simulink model "Prodline_EF_RL"  (R2023b)
settings: Solver=VariableStepDiscrete  StartTime=0  StopTime=Inf  RelTol=1e-3
model workspace (MAT data in the model file):
  EpisodeData.ExplorationProbability = 0.01
  EpisodeData.LearnRate = 0.7
  EpisodeData.DiscountFactor = 0.9
  EpisodeData.Table = [32.3279808057 48.3662273221 56.8010564606 75.8199870142 94.2467100891 126.392175074 147.868902265 201.713499215 225.197534088 273.928372258 470.902807484 558.602771343 ... (3844 elements, 1922x2)]
  EpisodeData.TotalReward = 0
  EpisodeData.LastEpisode = 0
  EpisodeData.Seed = 20000
  SimOptions.tMax = 480
  SimOptions.ProcessingTime_Job1 = 1
  SimOptions.ProcessingTime_Job2 = 3
  SimOptions.RetoolingTime = 3
  SimOptions.SaleTime_Job1 = 10
  SimOptions.SaleTime_Job2 = 5
  SimOptions.MaxQueueLength = 30
  SimOptions.MaxDeltaQueue = 10
undefined symbols (not defined in the file or in its folder): i, m, n
libraries: simulink x1, rllib x1
settings Model: SimulationMode=accelerator  Creator=jan  LastModifiedBy=jan
settings SolverCC: AllowMultiTaskInputOutput=on
settings OptimizationCC: ReuseModelBlockBuffer=off
settings ModelReferenceCC: EnableRefExpFcnMdlSchedulingChecks=on

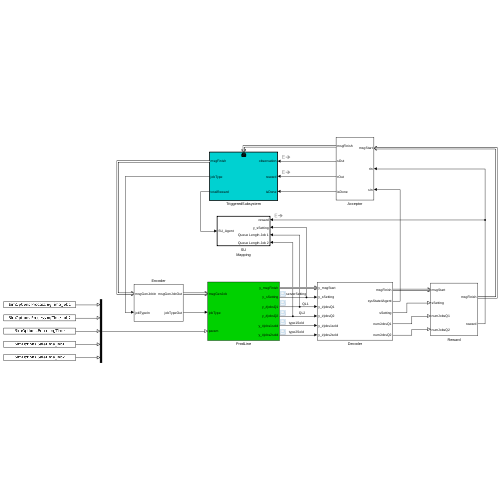
[thumbnail: Simulink's stored preview of the top-level diagram]
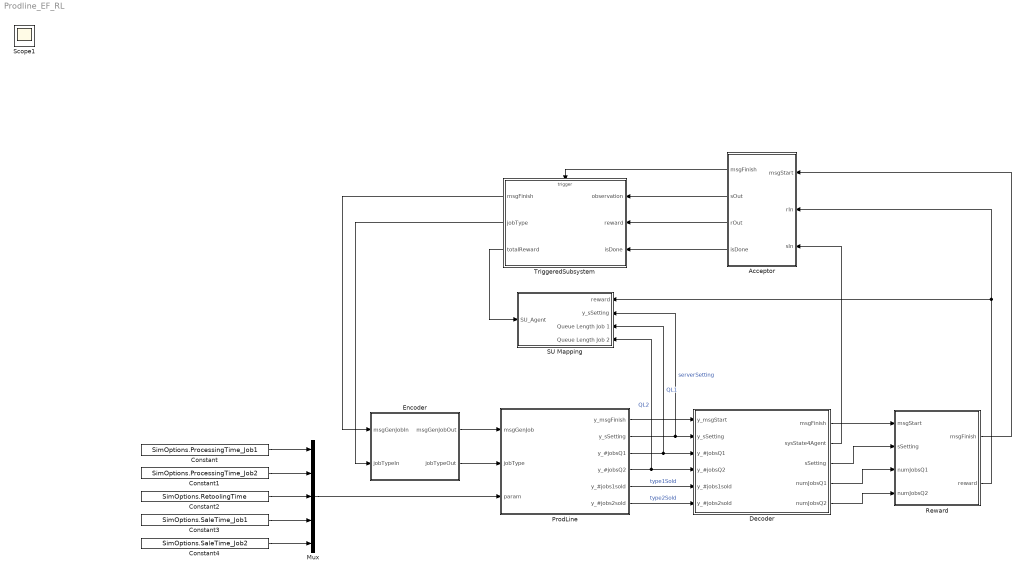
== system Prodline_EF_RL ==
  Acceptor : Subsystem
  Constant : Constant  Value=SimOptions.ProcessingTime_Job1
  Constant1 : Constant  Value=SimOptions.ProcessingTime_Job2
  Constant2 : Constant  Value=SimOptions.RetoolingTime
  Constant3 : Constant  Value=SimOptions.SaleTime_Job1
  Constant4 : Constant  Value=SimOptions.SaleTime_Job2
  Decoder : Subsystem
  Encoder : Subsystem
  Mux : Mux  Inputs=5
  ProdLine : Subsystem
  Reward : Subsystem
  SU Mapping : Subsystem  TreatAsAtomicUnit=on
      settings: PortSchema="{\"entries\":[{\"content\":{\"sides\":[{\"content\":{\"connectorIds\":[\"In1\",\"In2\",\"In3\",\"In4\"]},\"type\":\"ConnectorPlacement.EquallySpacedRectSide\",\"uuid\":\"25726879-9920-47f0-bc13-fe4ee4fad127\"},{\"content\":{\"connectorIds\":[\"In5\"],\"side\":\"RIGHT\"},\"type\":\"ConnectorPlacement.EquallySpacedRectSide\",\"uuid\":\"76e5ad88-c4d3-414b-b9a6-05d87e69b074\"},{\"content\":{\"connectorIds\":[],\"side\":\"TOP\"},\"type\":\"ConnectorPlacement.EquallySpacedRectSide\",\"uuid\":\"0e81be63-41e4-4d16-953c-cb60ef6ef114\"}]},\"type\":\"ConnectorPlacement.EquallySpacedConnector\",\"uuid\":\"9bcce8c0-ed31-4d29-947b-6e1387c3e550\"}],\"packageUris\":[\"http://schema.mathworks.com/mf0/Connector/R2020b\"],\"version\":\"1.0\"}"
  TriggeredSubsystem : Subsystem  InputPortMessageModes=i,i,i,m  TreatAsAtomicUnit=on
  Scope1 : Scope
  wires:
  Mux/1 -> ProdLine/3(param)
  Constant/1 -> Mux/1
  Constant1/1 -> Mux/2
  Constant2/1 -> Mux/3
  Constant3/1 -> Mux/4
  Constant4/1 -> Mux/5
  Encoder/1(msgGenJobOut) -> ProdLine/1(msgGenJob)
  Encoder/2(jobTypeOut) -> ProdLine/2(jobType)
  ProdLine/2(y_sSetting) -> Decoder/2(y_sSetting), SU Mapping/2(y_sSetting)  "serverSetting"
  ProdLine/3(y_#jobsQ1) -> SU Mapping/3(Queue Length Job 1), Decoder/3(y_#jobsQ1)  "QL1"
  ProdLine/4(y_#jobsQ2) -> Decoder/4(y_#jobsQ2), SU Mapping/4(Queue Length Job 2)  "QL2"
  ProdLine/5(y_#jobs1sold) -> Decoder/5(y_#jobs1sold)  "type1Sold"
  ProdLine/6(y_#jobs2sold) -> Decoder/6(y_#jobs2sold)  "type2Sold"
  Decoder/1(msgFinish) -> Reward/1(msgStart)
  ProdLine/1(y_msgFinish) -> Decoder/1(y_msgStart)
  Decoder/3(sSetting) -> Reward/2(sSetting)
  Decoder/4(numJobsQ1) -> Reward/3(numJobsQ1)
  Decoder/5(numJobsQ2) -> Reward/4(numJobsQ2)
  Decoder/2(sysState4Agent) -> Acceptor/3(sIn)
  Reward/1(msgFinish) -> Acceptor/1(msgStart)
  Reward/2(reward) -> SU Mapping/1(reward), Acceptor/2(rIn)
  Acceptor/3(rOut) -> TriggeredSubsystem/2(reward)
  Acceptor/4(isDone) -> TriggeredSubsystem/3(isDone)
  Acceptor/1(msgFinish) -> TriggeredSubsystem/Trigger
  TriggeredSubsystem/1(msgFinish) -> Encoder/1(msgGenJobIn)
  TriggeredSubsystem/2(jobType) -> Encoder/2(jobTypeIn)
  TriggeredSubsystem/3(totalReward) -> SU Mapping/5(SU_Agent)
  Acceptor/2(sOut) -> TriggeredSubsystem/1(observation)

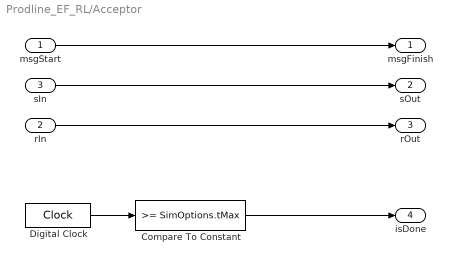
== system Prodline_EF_RL/Acceptor ==
  msgStart : Inport
  rIn : Inport  Port=2
  sIn : Inport  Port=3
  Compare To Constant : simulink/Logic and Bit Operations/Compare To Constant  relop=>=  const=SimOptions.tMax  OutDataTypeStr=boolean  ZeroCross=off
  Digital Clock : DigitalClock
  msgFinish : Outport
  sOut : Outport  Port=2
  rOut : Outport  Port=3
  isDone : Outport  Port=4
  wires:
  Digital Clock/1 -> Compare To Constant/1
  sIn/1 -> sOut/1
  msgStart/1 -> msgFinish/1
  rIn/1 -> rOut/1
  Compare To Constant/1 -> isDone/1

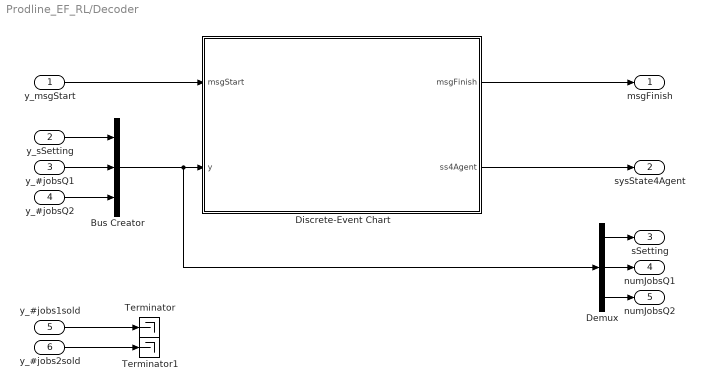
== system Prodline_EF_RL/Decoder ==
  y_msgStart : Inport
  y_sSetting : Inport  Port=2
  y_#jobsQ1 : Inport  Port=3
  y_#jobsQ2 : Inport  Port=4
  y_#jobs1sold : Inport  Port=5
  y_#jobs2sold : Inport  Port=6
  Bus Creator : BusCreator  Inputs=3
  Demux : Demux  Outputs=3
  Discrete-Event Chart : Stateflow chart  TreatAsAtomicUnit=on
  Terminator : Terminator
  Terminator1 : Terminator
  msgFinish : Outport
  sysState4Agent : Outport  Port=2  OutDataTypeStr=uint32
  sSetting : Outport  Port=3
  numJobsQ1 : Outport  Port=4
  numJobsQ2 : Outport  Port=5
  wires:
  Discrete-Event Chart/2(ss4Agent) -> sysState4Agent/1
  Bus Creator/1 -> Demux/1, Discrete-Event Chart/2(y)
  y_sSetting/1 -> Bus Creator/1
  y_#jobsQ1/1 -> Bus Creator/2
  y_#jobsQ2/1 -> Bus Creator/3
  Discrete-Event Chart/1(msgFinish) -> msgFinish/1
  y_#jobs1sold/1 -> Terminator/1
  y_#jobs2sold/1 -> Terminator1/1
  Demux/2 -> numJobsQ1/1
  Demux/1 -> sSetting/1
  Demux/3 -> numJobsQ2/1
  y_msgStart/1 -> Discrete-Event Chart/1(msgStart)

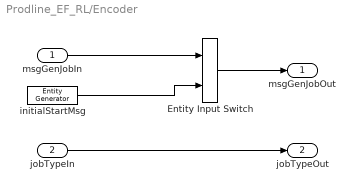
== system Prodline_EF_RL/Encoder ==
  msgGenJobIn : Inport
  jobTypeIn : Inport  Port=2
  Entity Input Switch : EntityInputSwitch  InputPortMessageModes=m,m  OutputPortMessageModes=m
  initialStartMsg : EntityGenerator  OutputPortMessageModes=m  Period=Inf  AttributeName=entity  EntityTypeName=Entity  DataInitialValue=1
  msgGenJobOut : Outport
  jobTypeOut : Outport  Port=2
  wires:
  msgGenJobIn/1 -> Entity Input Switch/1
  initialStartMsg/1 -> Entity Input Switch/2
  Entity Input Switch/1 -> msgGenJobOut/1
  jobTypeIn/1 -> jobTypeOut/1

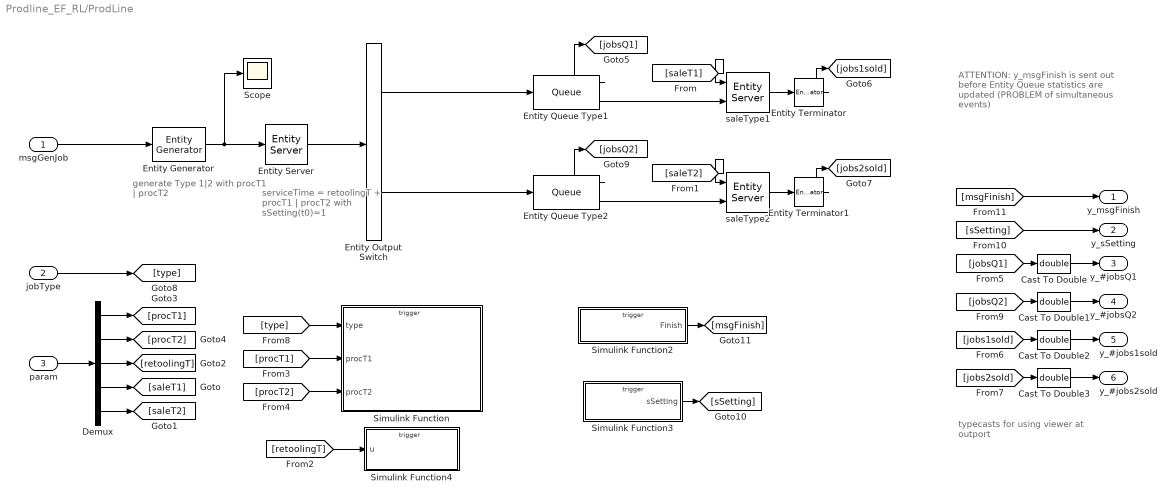
== system Prodline_EF_RL/ProdLine ==
  note: generate Type 1|2
      | with procT1 | procT2
  note: ATTENTION:
      | y_msgFinish is sent out
      | before Entity Queue
      | statistics are updated
      | (PROBLEM of
      | simultaneous events)
  note: serviceTime =
      | retoolingT +
      | procT1 | procT2
      |      with
      | sSetting(t0)=1
  note: typecasts for using
      | viewer at outport
  msgGenJob : Inport
  jobType : Inport  Port=2
  param : Inport  Port=3
  Cast To Double{,1..3} (4 alike) : DataTypeConversion  OutDataTypeStr=double  SaturateOnIntegerOverflow=off  RndMeth=Floor
  Demux : Demux  Outputs=5
  Entity Output Switch : EntityOutputSwitch  InputPortMessageModes=m  OutputPortMessageModes=m,m  SwitchingCriterion=From attribute  SwitchAttributeName=Type
  Entity Generator : EntityGenerator  InputPortMessageModes=m  OutputPortMessageModes=m  GenerationMethod=Event-based  GenerateAction=|  AttributeName=ID|Type|ProcessingTime|ServiceTime  AttributeInitialValue=1|0|0|0  EntityType=Structured  EntityTypeName=Job
      | % Use a persistent counter to set ID
      | persistent next_id
      | if isempty(next_id)
      |     next_id = 1;
      |     %{
      |     % IS NOT Necessary!
      |     % Set seed for random number generator
      |     rng(12345)
      |     %}
      | end
      | 
      | % Assign ID attribute
      | entity.ID = next_id;
      | next_id = next_id +1;
      | 
      | %Assign job Type and ProcessingTime
      | %entity.Type = setJobType()
      | [entity.Type,entity.ProcessingTime]=setAttributes();
      settings: InputPortMap=u0
  Entity Queue Type1 : Queue  InputPortMessageModes=m  OutputPortMessageModes=n,m  Capacity=Inf  EntryAction=|  NumberEntitiesInBlock=on
      | % Generate finish msg
      | sendFinish(entity.Type)
      settings: OutputPortMap=o1,o5
  Entity Queue Type2 : Queue  InputPortMessageModes=m  OutputPortMessageModes=n,m  Capacity=Inf  EntryAction=|  NumberEntitiesInBlock=on
      | % Generate finish msg
      | sendFinish(entity.Type);
      settings: OutputPortMap=o1,o5
  Entity Server : EntityServer  InputPortMessageModes=m  OutputPortMessageModes=m  Capacity=1  ServiceTimeSource=Attribute  EntryAction=|  ExitAction=|
      EntryAction=|
      | % Use a persistent var to store the current server setting
      | % server setting is 1 | 2
      | persistent serverSetting
      | if isempty(serverSetting)
      |     serverSetting = 1;     % init serverSetting
      | end
      | 
      | % Test if new serverSetting is necessary (retooling)
      | if serverSetting ~= entity.Type
      |    entity.ServiceTime = entity.ProcessingTime + retoolingTime();
      |    serverSetting = entity.Type;
      | else
      |     entity.ServiceTime = entity.ProcessingTime;
      | end
      | 
      | % Output current serverSetting
      | outServerSetting(serverSetting)
      ExitAction=|
      | % Generate finish msg
      | %sendFinish();
  Entity Terminator : EntityTerminator  InputPortMessageModes=m  NumberEntitiesArrived=on
      settings: OutputPortMap=o0
  Entity Terminator1 : EntityTerminator  InputPortMessageModes=m  NumberEntitiesArrived=on
      settings: OutputPortMap=o0
  Scope : Scope
  Simulink Function : Subsystem  TreatAsAtomicUnit=on
  Simulink Function2 : Subsystem  TreatAsAtomicUnit=on
  Simulink Function3 : Subsystem  TreatAsAtomicUnit=on
  Simulink Function4 : Subsystem  TreatAsAtomicUnit=on
  saleType1 : EntityServer  InputPortMessageModes=n,m  OutputPortMessageModes=m  Capacity=1  ServiceTimeSource=Signal port  ServiceTimeValue=10
      settings: InputPortMap=u0,u2
  saleType2 : EntityServer  InputPortMessageModes=n,m  OutputPortMessageModes=m  Capacity=1  ServiceTimeSource=Signal port  ServiceTimeValue=5
      settings: InputPortMap=u0,u2
  y_msgFinish : Outport
  y_sSetting : Outport  Port=2
  y_#jobsQ1 : Outport  Port=3
  y_#jobsQ2 : Outport  Port=4
  y_#jobs1sold : Outport  Port=5
  y_#jobs2sold : Outport  Port=6
  wires:
  Simulink Function2/1(" Finish") -> [msgFinish]
  [procT2] -> Simulink Function/3(procT2)
  Demux/5 -> [saleT2]
  Entity Terminator1/1 -> [jobs2sold]
  Entity Output Switch/1 -> Entity Queue Type1/1
  [jobs2sold] -> Cast To Double3/1
  Demux/2 -> [procT2]
  Simulink Function3/1(sSetting) -> [sSetting]
  Cast To Double2/1 -> y_#jobs1sold/1
  [saleT1] -> saleType1/1
  [jobsQ2] -> Cast To Double1/1
  [retoolingT] -> Simulink Function4/1(u)
  Cast To Double3/1 -> y_#jobs2sold/1
  [type] -> Simulink Function/1(type)
  [msgFinish] -> y_msgFinish/1
  Entity Server/1 -> Entity Output Switch/1
  Entity Generator/1 -> Scope/1, Entity Server/1
  Demux/1 -> [procT1]
  Entity Output Switch/2 -> Entity Queue Type2/1
  jobType/1 -> [type]
  param/1 -> Demux/1
  Demux/4 -> [saleT1]
  Entity Terminator/1 -> [jobs1sold]
  [procT1] -> Simulink Function/2(procT1)
  Cast To Double1/1 -> y_#jobsQ2/1
  msgGenJob/1 -> Entity Generator/1
  Entity Queue Type2/2 -> saleType2/2
  [jobsQ1] -> Cast To Double/1
  Entity Queue Type1/2 -> saleType1/2
  Demux/3 -> [retoolingT]
  Entity Queue Type1/1 -> [jobsQ1]
  Cast To Double/1 -> y_#jobsQ1/1
  [saleT2] -> saleType2/1
  [sSetting] -> y_sSetting/1
  saleType1/1 -> Entity Terminator/1
  Entity Queue Type2/1 -> [jobsQ2]
  saleType2/1 -> Entity Terminator1/1
  [jobs1sold] -> Cast To Double2/1

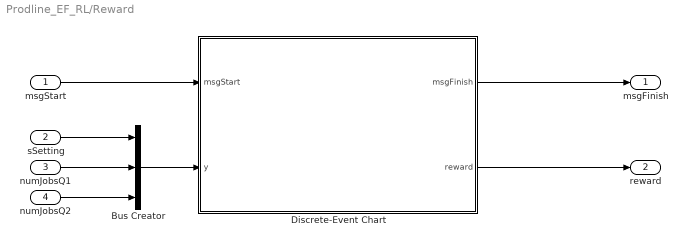
== system Prodline_EF_RL/Reward ==
  msgStart : Inport
  sSetting : Inport  Port=2
  numJobsQ1 : Inport  Port=3
  numJobsQ2 : Inport  Port=4
  Bus Creator : BusCreator  Inputs=3
  Discrete-Event Chart : Stateflow chart  TreatAsAtomicUnit=on
  msgFinish : Outport
  reward : Outport  Port=2
  wires:
  Discrete-Event Chart/1(msgFinish) -> msgFinish/1
  msgStart/1 -> Discrete-Event Chart/1(msgStart)
  Discrete-Event Chart/2(reward) -> reward/1
  Bus Creator/1 -> Discrete-Event Chart/2(y)
  numJobsQ1/1 -> Bus Creator/2
  sSetting/1 -> Bus Creator/1
  numJobsQ2/1 -> Bus Creator/3

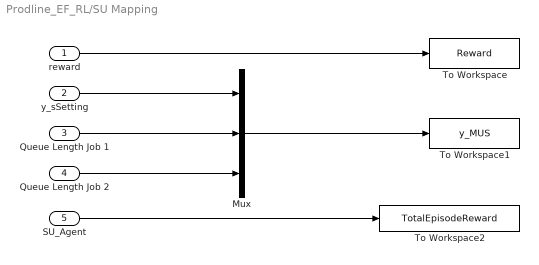
== system Prodline_EF_RL/SU Mapping ==
  reward : Inport
  y_sSetting : Inport  Port=2
  Queue Length Job 1 : Inport  Port=3
  Queue Length Job 2 : Inport  Port=4
  SU_Agent : Inport  Port=5
  Mux : Mux  Inputs=3
  To Workspace : ToWorkspace  VariableName=Reward  SaveFormat=Timeseries  SampleTime=-1
  To Workspace1 : ToWorkspace  VariableName=y_MUS  SaveFormat=Timeseries  SampleTime=-1
  To Workspace2 : ToWorkspace  VariableName=TotalEpisodeReward  SaveFormat=Timeseries  SampleTime=-1
      settings: MaxDataPoints=1
  wires:
  reward/1 -> To Workspace/1
  y_sSetting/1 -> Mux/1
  Queue Length Job 1/1 -> Mux/2
  Queue Length Job 2/1 -> Mux/3
  Mux/1 -> To Workspace1/1
  SU_Agent/1 -> To Workspace2/1

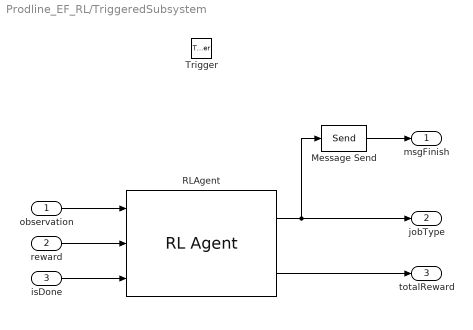
== system Prodline_EF_RL/TriggeredSubsystem ==
  observation : Inport
  reward : Inport  Port=2
  isDone : Inport  Port=3
  Trigger : TriggerPort  TriggerType=message  ScheduleAsAperiodic=off  FunctionName=TriggeredSubsystem  FunctionVisibility=scoped  VariantControl=(inherit)
  Message Send : Send  OutputPortMessageModes=m
  RLAgent : rllib/RL Agent  Agent=Agent  ExternalActionAsInput=off  ProvideLastAction=off  ProvideCumRwd=on  TreatAsDirectFeedthrough=on  UseStrictObservationDataTypes=off
  msgFinish : Outport
  jobType : Outport  Port=2  InitialOutput=[1]
  totalReward : Outport  Port=3
  wires:
  observation/1 -> RLAgent/1
  reward/1 -> RLAgent/2
  isDone/1 -> RLAgent/3
  RLAgent/1 -> Message Send/1, jobType/1
  RLAgent/2 -> totalReward/1
  Message Send/1 -> msgFinish/1

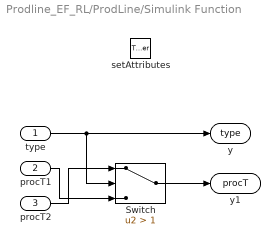
== system Prodline_EF_RL/ProdLine/Simulink Function ==
  type : Inport
  procT1 : Inport  Port=2
  procT2 : Inport  Port=3
  setAttributes : TriggerPort  TriggerType=function-call  IsSimulinkFunction=on  FunctionName=setAttributes  FunctionVisibility=scoped  VariantControl=Variant
  Switch : Switch  Criteria=u2 > Threshold  Threshold=1  SaturateOnIntegerOverflow=off  InputSameDT=off
  y : ArgOut  DisableCoverage=on  ArgumentName=type
  y1 : ArgOut  DisableCoverage=on  Port=2  ArgumentName=procT
  wires:
  type/1 -> Switch/2, y/1
  Switch/1 -> y1/1
  procT2/1 -> Switch/1
  procT1/1 -> Switch/3

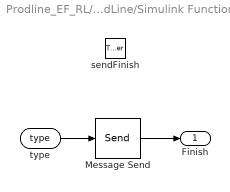
== system Prodline_EF_RL/ProdLine/Simulink Function2 ==
  sendFinish : TriggerPort  TriggerType=function-call  IsSimulinkFunction=on  FunctionName=sendFinish  FunctionVisibility=scoped  VariantControl=(inherit)
  Message Send : Send  OutputPortMessageModes=m
  type : ArgIn  DisableCoverage=on  ArgumentName=type
  " Finish" : Outport
  wires:
  Message Send/1 -> " Finish"/1
  type/1 -> Message Send/1

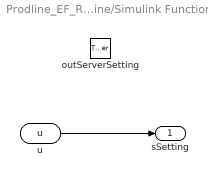
== system Prodline_EF_RL/ProdLine/Simulink Function3 ==
  outServerSetting : TriggerPort  TriggerType=function-call  IsSimulinkFunction=on  FunctionName=outServerSetting  FunctionVisibility=scoped  VariantControl=(inherit)
  u : ArgIn  DisableCoverage=on  ArgumentName=u
  sSetting : Outport
  wires:
  u/1 -> sSetting/1

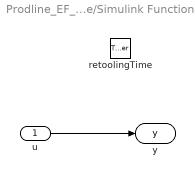
== system Prodline_EF_RL/ProdLine/Simulink Function4 ==
  u : Inport
  retoolingTime : TriggerPort  TriggerType=function-call  IsSimulinkFunction=on  FunctionName=retoolingTime  FunctionVisibility=scoped  VariantControl=Variant
  y : ArgOut  DisableCoverage=on  ArgumentName=y
  wires:
  u/1 -> y/1

== stateflow chart Prodline_EF_RL/Reward/Discrete-Event Chart ==
  settings: enableNonTerminalStates=1
  state wait
  state getState4Agent
    en:
    reward = getReward(y(2),y(3));
    send(msgFinish);
  (default) -> wait : {msgFinish.data=1;}
  wait -> getState4Agent : msgStart
  getState4Agent -> wait
  data: ql1 function_input; ql2 function_input; r function_output; msgStart input; y input; msgFinish output; reward output
  function r = getReward(ql1, ql2):
    | function r = getReward(ql1, ql2)
    |     
    |     if ql1 >= 10 && ql2 >= 10
    |         r = 100;
    |     elseif ql1 >=10
    |         r = ql2^2;
    |     elseif ql2 >=10
    |         r = ql1^2;
    |     else
    |         r = ((ql2)^2*(ql1)^2)/100;
    |     end
    | end

== stateflow chart Prodline_EF_RL/Decoder/Discrete-Event Chart ==
  settings: enableNonTerminalStates=1
  note: wait a short amount of time to get the updated queue lengths from the production line model
  state updateDelay
  state wait
  state getState4Agent
    en:
    ss4Agent = obs2State(y(1),y(2),y(3));
    send(msgFinish);
  (default) -> wait : {msgFinish.data=1;}
  wait -> updateDelay : msgStart
  updateDelay -> getState4Agent : after(1e-6,'sec')
  getState4Agent -> wait
  data: y_JType function_input; y_QL1 function_input; y_QL2 function_input; sysState4Agent function_output; msgStart input; y input; msgFinish output; ss4Agent output =uint32(1); EpisodeData parameter; SimOptions parameter
  function sysState4Agent = obs2State(y_JType, y_QL1, y_QL2):
    | function sysState4Agent = obs2State(y_JType, y_QL1, y_QL2)
    |     
    | persistent stateSpaceSize queueLengthMax;
    | 
    | if isempty(stateSpaceSize)
    |     stateSpaceSize = size(EpisodeData.Table, 1);
    |     queueLengthMax = SimOptions.MaxQueueLength;
    | end
    | 
    | % limit queue lenght to stay in state space
    | y_QL1 = min(y_QL1, queueLengthMax);
    | y_QL2 = min(y_QL2, queueLengthMax);
    | 
    | % encode the three states to a unique RL-state
    | sysState4Agent = uint32( ...
    |     (y_JType-1) * (queueLengthMax+1)^2 + ...
    |     y_QL1 * (queueLengthMax+1) + y_QL2 + 1);
    | 
    | end
